simulink model "Vertical_rolling_Tongji_Model"  (R2021b)
settings: Solver=ode23s  StartTime=0.0  StopTime=7.5  FixedStep=1e-3  MaxStep=1e-3  RelTol=1e-3
values from neighbouring files (symbols this model uses):
  J_1 = m_1*r_1^2/2    (= 0.1)    [Vertical_Rolling_Tongji.m]
  J_2 = m_2*r_2^2/2    (= 2.5)    [Vertical_Rolling_Tongji.m]
  m_1 = 5    [Vertical_Rolling_Tongji.m]
  m_2 = 20    [Vertical_Rolling_Tongji.m]
  mu_d = 0.5    [Vertical_Rolling_Tongji.m]
  mu_r = mu_s*10^-2    (= 0.0065)    [Vertical_Rolling_Tongji.m]
  mu_s = 0.65    [Vertical_Rolling_Tongji.m]
  r_1 = 0.2    [Vertical_Rolling_Tongji.m]
  r_2 = 0.5    [Vertical_Rolling_Tongji.m]
libraries: simulink x4
settings Model: Creator=Gioele  LastModifiedBy=gioele
settings SolverCC: AlgebraicLoopSolver=TrustRegion
settings DebuggingCC: AlgebraicLoopMsg=none  SFMachineParentedDataDiag=warning

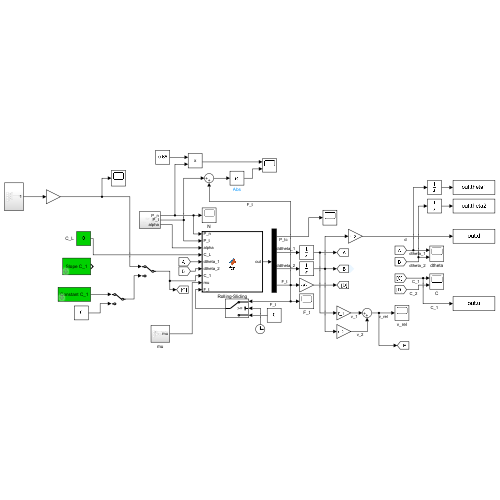
[thumbnail: Simulink's stored preview of the top-level diagram]
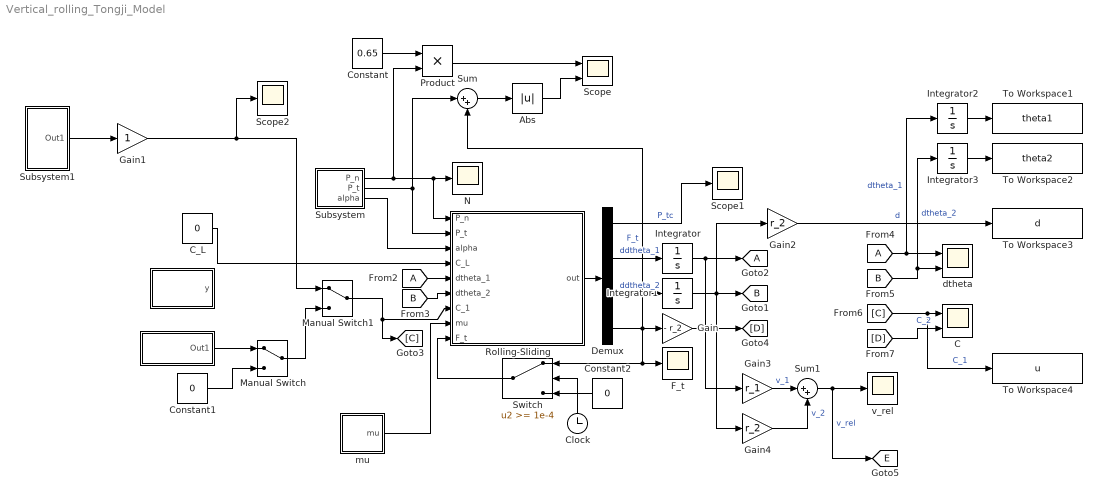
== system Vertical_rolling_Tongji_Model ==
  " " : Subsystem  mask{C_1_slope_gain=1.0}
      mask prompts: C_1_slope_gain "Slope C_1 gain"
      mask Display: disp('Slope C_1')
  "  " : Subsystem  mask{C_1_constant=0}
      mask prompts: C_1_constant "Constant C_1"
      mask Display: disp('Constant C_1')
  Abs : Abs
  C : Scope  NumInputPorts=2
  C_L : Constant  Value=0
  Clock : Clock
  Constant : Constant  Value=0.65
  Constant1 : Constant  Value=0
  Constant2 : Constant  Value=0
  Demux : Demux
  F_t : Scope
  Gain : Gain  Gain=- r_2
  Gain1 : Gain
  Gain2 : Gain  Gain=r_2
  Gain3 : Gain  Gain=r_1
  Gain4 : Gain  Gain=r_2
  Integrator{,1..3} (4 alike) : Integrator
  Manual Switch : ManualSwitch
  Manual Switch1 : ManualSwitch
  N : Scope
  Product : Product
  Rolling-Sliding : MATLAB Function  TreatAsAtomicUnit=on
  Scope : Scope  NumInputPorts=2
  Scope1 : Scope
  Scope2 : Scope
  Subsystem : Subsystem
  Subsystem1 : Subsystem
  Sum : Sum  Inputs=|++
  Sum1 : Sum  Inputs=|++
  Switch : Switch  Threshold=1e-4
  To Workspace1 : ToWorkspace  VariableName=theta1  SampleTime=1e-2
  To Workspace2 : ToWorkspace  VariableName=theta2  SampleTime=1e-2
  To Workspace3 : ToWorkspace  VariableName=d  SampleTime=1e-2
  To Workspace4 : ToWorkspace  VariableName=u  SampleTime=1e-2
  dtheta : Scope  NumInputPorts=2
  mu : Subsystem
  v_rel : Scope
  tag scope: A=global, B=global, E=global
  wires:
  Demux/2 -> Integrator/1  "ddtheta_1"
  Gain3/1 -> Sum1/1  "v_1"
  Gain4/1 -> Sum1/2  "v_2"
  Constant2/1 -> Switch/3
  Clock/1 -> Switch/2
  [A] -> Rolling-Sliding/5(dtheta_1)
  Manual Switch1/1 -> [C], Rolling-Sliding/7(C_1)
  Integrator/1 -> [A], Gain3/1
  [B] -> Rolling-Sliding/6(dtheta_2)
  Sum1/1 -> [E], v_rel/1  "v_rel"
  Manual Switch/1 -> Manual Switch1/2
  Constant1/1 -> Manual Switch/2
  Demux/3 -> Integrator1/1  "ddtheta_2"
  Integrator1/1 -> Gain2/1, [B], Gain4/1
  Rolling-Sliding/1(out) -> Demux/1
  Demux/4 -> Sum/2, F_t/1, Switch/1, Gain/1  "F_t"
  Gain/1 -> [D]
  Switch/1 -> Rolling-Sliding/9(F_t)
  C_L/1 -> Rolling-Sliding/4(C_L)
  "  "/1(Out1) -> Manual Switch/1
  mu/1(mu) -> Rolling-Sliding/8(mu)
  Subsystem/1(P_n) -> Product/2, Rolling-Sliding/1(P_n), N/1
  Integrator2/1 -> To Workspace1/1
  [A] -> Integrator2/1, dtheta/1  "dtheta_1"
  [B] -> Integrator3/1, dtheta/2  "dtheta_2"
  Integrator3/1 -> To Workspace2/1
  Subsystem/2(P_t) -> Rolling-Sliding/2(P_t), Sum/1
  Sum/1 -> Abs/1
  Constant/1 -> Product/1
  Product/1 -> Scope/1
  Abs/1 -> Scope/2
  Demux/1 -> Scope1/1  "P_tc"
  Subsystem/3(alpha) -> Rolling-Sliding/3(alpha)
  Gain1/1 -> Scope2/1, Manual Switch1/1
  Subsystem1/1(Out1) -> Gain1/1
  [D] -> C/2  "C_2"
  [C] -> To Workspace4/1, C/1  "C_1"
  Gain2/1 -> To Workspace3/1  "d"

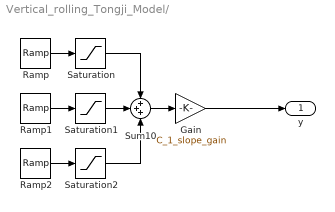
== system Vertical_rolling_Tongji_Model/  ==
  Gain : Gain  Gain=C_1_slope_gain
  Ramp : simulink/Sources/Ramp  slope=1  start=5  InitialOutput=0
  Ramp1 : simulink/Sources/Ramp  slope=1  start=15  InitialOutput=0
  Ramp2 : simulink/Sources/Ramp  slope=-1  start=25  InitialOutput=0
  Saturation : Saturate  UpperLimit=5  LowerLimit=0
  Saturation1 : Saturate  UpperLimit=5  LowerLimit=0
  Saturation2 : Saturate  UpperLimit=0  LowerLimit=-10
  Sum10 : Sum  Inputs=+++
  y : Outport
  wires:
  Saturation1/1 -> Sum10/2
  Sum10/1 -> Gain/1
  Ramp1/1 -> Saturation1/1
  Saturation/1 -> Sum10/1
  Ramp2/1 -> Saturation2/1
  Ramp/1 -> Saturation/1
  Gain/1 -> y/1
  Saturation2/1 -> Sum10/3

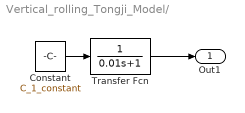
== system Vertical_rolling_Tongji_Model/   ==
  Constant : Constant  Value=C_1_constant
  Transfer Fcn : TransferFcn  Denominator=[0.01 1]
  Out1 : Outport
  wires:
  Constant/1 -> Transfer Fcn/1
  Transfer Fcn/1 -> Out1/1

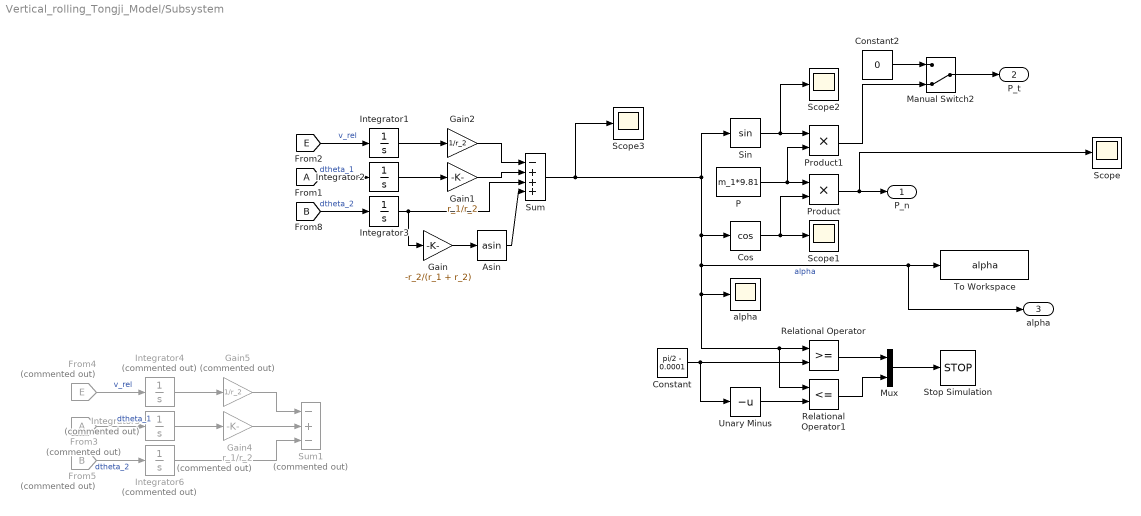
== system Vertical_rolling_Tongji_Model/Subsystem ==
  Asin : Trigonometry  Operator=asin
  Constant : Constant  Value=pi/2 - 0.0001
  Constant2 : Constant  Value=0
  Cos : Trigonometry  Operator=cos
  From3 : From  Commented=on  TagVisibility=global
  From4 : From  Commented=on  GotoTag=E  TagVisibility=global
  From5 : From  Commented=on  GotoTag=B  TagVisibility=global
  Gain : Gain  Gain=-r_2/(r_1 + r_2)
  Gain1 : Gain  Gain=r_1/r_2
  Gain2 : Gain  Gain=1/r_2
  Gain4 : Gain  Commented=on  Gain=r_1/r_2
  Gain5 : Gain  Commented=on  Gain=1/r_2
  Integrator1 : Integrator
  Integrator2 : Integrator
  Integrator3 : Integrator
  Integrator4 : Integrator  Commented=on
  Integrator5 : Integrator  Commented=on
  Integrator6 : Integrator  Commented=on
  Manual Switch2 : ManualSwitch  CurrentSetting=0
  Mux : Mux  Inputs=2
  P : Constant  Value=m_1*9.81
  Product : Product
  Product1 : Product
  Relational Operator : RelationalOperator  OutDataTypeStr=boolean  RndMeth=Simplest
  Relational Operator1 : RelationalOperator  Operator=<=  OutDataTypeStr=boolean  RndMeth=Simplest
  Scope{,1..3} (4 alike) : Scope
  Sin : Trigonometry
  Stop Simulation : Stop
  Sum : Sum  Inputs=-+++
  Sum1 : Sum  Commented=on  Inputs=-+-
  To Workspace : ToWorkspace  VariableName=alpha  SampleTime=1e-2
  Unary Minus : UnaryMinus
  "alpha " : Scope
  P_n : Outport
  P_t : Outport  Port=2
  alpha : Outport  Port=3
  wires:
  P/1 -> Product1/2, Product/1
  [A] -> Integrator2/1  "dtheta_1"
  Integrator3/1 -> Sum/3, Gain/1
  Integrator2/1 -> Gain1/1
  [B] -> Integrator3/1  "dtheta_2"
  Product/1 -> Scope/1, P_n/1
  Gain1/1 -> Sum/2
  Cos/1 -> Scope1/1, Product/2
  Sum/1 -> Cos/1, Relational Operator1/1, Relational Operator/1, "alpha "/1, alpha/1, To Workspace/1, Sin/1, Scope3/1  "alpha"
  Gain/1 -> Asin/1
  [E] -> Integrator1/1  "v_rel"
  Integrator1/1 -> Gain2/1
  Gain2/1 -> Sum/1
  Constant/1 -> Unary Minus/1, Relational Operator/2
  Unary Minus/1 -> Relational Operator1/2
  Relational Operator/1 -> Mux/1
  Relational Operator1/1 -> Mux/2
  Mux/1 -> Stop Simulation/1
  Sin/1 -> Scope2/1, Product1/1
  Product1/1 -> Manual Switch2/2
  Constant2/1 -> Manual Switch2/1
  Manual Switch2/1 -> P_t/1
  Asin/1 -> Sum/4
  From5/1 -> Integrator6/1  "dtheta_2"
  Gain5/1 -> Sum1/1
  Integrator5/1 -> Gain4/1
  Gain4/1 -> Sum1/2
  Integrator4/1 -> Gain5/1
  Integrator6/1 -> Sum1/3
  From4/1 -> Integrator4/1  "v_rel"
  From3/1 -> Integrator5/1  "dtheta_1"

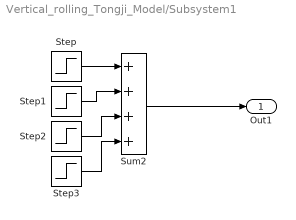
== system Vertical_rolling_Tongji_Model/Subsystem1 ==
  Step : Step  After=0.5  SampleTime=0
  Step1 : Step  Time=2  After=-1.5  SampleTime=0
  Step2 : Step  Time=3  After=3  SampleTime=0
  Step3 : Step  Time=4  After=-4  SampleTime=0
  Sum2 : Sum  Inputs=++++
  Out1 : Outport
  wires:
  Step2/1 -> Sum2/3
  Step1/1 -> Sum2/2
  Sum2/1 -> Out1/1
  Step3/1 -> Sum2/4
  Step/1 -> Sum2/1

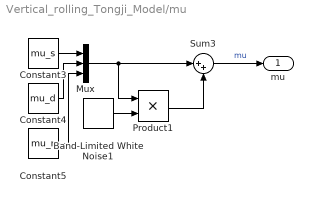
== system Vertical_rolling_Tongji_Model/mu ==
  Band-Limited White Noise1 : simulink/Sources/Band-Limited White Noise  Cov=[0.000001]  Ts=0.1  seed=[23341]
  Constant3 : Constant  Value=mu_s
  Constant4 : Constant  Value=mu_d
  Constant5 : Constant  Value=mu_r
  Mux : Mux  Inputs=3
  Product1 : Product
  Sum3 : Sum  Inputs=|++
  mu : Outport
  wires:
  Sum3/1 -> mu/1  "mu"
  Constant5/1 -> Mux/3
  Band-Limited White Noise1/1 -> Product1/2
  Constant4/1 -> Mux/2
  Product1/1 -> Sum3/2
  Constant3/1 -> Mux/1
  Mux/1 -> Sum3/1, Product1/1

== matlab function Vertical_rolling_Tongji_Model/Rolling-Sliding ==
  data: P_n input; P_t input; alpha input; C_L input; dtheta_1 input; dtheta_2 input; C_1 input; r_1 parameter; r_2 parameter; J_1 parameter; J_2 parameter; mu input; F_t input; out output; m_2 parameter
function out = fcn(P_n,P_t,alpha,C_L,dtheta_1,dtheta_2,C_1,r_1,r_2,J_1,J_2,mu,F_t, m_2)
% Define the inputs of the function, some will be variables coming from the
% system, others will be parametsr from the workspace

mu_s_n = mu(1);
mu_d_n = mu(2);
mu_r_n = mu(3);
% Extract the values for the coefficients of friction from the white noise
% simulator

if abs(dtheta_1) > 0.01
    C_rf1 = - sign(dtheta_1)*mu_r_n*P_n;
else
    if abs(C_1) < mu_r_n*P_n
        C_rf1 = - C_1;
    else
        C_rf1 = - sign(dtheta_1)*mu_r_n*P_n;
    end
end
if abs(dtheta_2) > 0.01
    C_rf2 = - sign(dtheta_2)*mu_r_n*P_n;
else
    if abs(- F_t*r_2) < mu_r_n*P_n
        C_rf2 = - (- F_t*r_2);
    else
        C_rf2 = - sign(dtheta_2)*mu_r_n*P_n;
    end
end
% Define the action of the rolling friction forces C_rf1 and C_rf2

if (-0.0001 < dtheta_1*r_1 + dtheta_2*r_2) && (dtheta_1*r_1 + dtheta_2*r_2 < 0.0001)
    % Condition should be (dtheta_1*r_1 + dtheta_2*r_2 == 0) but need
    % tolerance for simulation reasons
    P_tc = P_t;
    F_t = (C_1*(r_1/J_1) + C_rf1*(r_1/J_1) + C_rf2*(r_2/J_2) + C_L*J_1*r_2 - P_tc*(r_1^2/J_1) - P_tc*(r_2^2/J_2) - P_n*sin(alpha)*(r_2^2/(J_2+m_2*r_2^2)))/((r_1^2/J_1) + (r_2^2/J_2));
    % Define the two tangential forces P_tc and F_t in the pure rolling
    % case
    if (abs(F_t + P_tc) > mu_s_n*P_n)
        P_tc = sign(alpha)*mu_d_n*P_n;
        F_t = sign(dtheta_1*r_1 + dtheta_2*r_2)*mu_d_n*P_n;
        % Transition from Rolling to Rolling with sliding
    end
else
    P_tc = sign(alpha)*mu_d_n*P_n;
    F_t = sign(dtheta_1*r_1 + dtheta_2*r_2)*mu_d_n*P_n;
    % Define the two tangential forces P_tc and F_t in the pure rolling
    % case
end

ddtheta_1 = (C_1 + C_rf1 - F_t*r_1 - P_tc*r_1)/(J_1);
ddtheta_2 = ((- F_t*r_2 - P_tc*r_2 + C_rf2 )/(J_2))-((P_n*sin(alpha)*r_2)/(J_2+m_2*r_2^2));
% Get out the final expression for the two angular speeds

out = [P_tc,ddtheta_1,ddtheta_2,F_t];
% Define the outputs of the system
